simulink model "lab3Koshi"
settings: Solver=ode45  StartTime=0.0  StopTime=100  RelTol=1e-3
libraries: simulink x2
settings Model: Creator=Шландаков  LastModifiedBy=Mihail
settings DataIOCC: LimitDataPoints=on  SaveFormat=Array  ReturnWorkspaceOutputs=off
settings OptimizationCC: LifeSpan=inf  SimCompilerOptimization=Off
settings DebuggingCC: UnderspecifiedInitializationDetection=Classic  MergeDetectMultiDrivingBlocksExec=none  SolverPrmCheckMsg=warning  MultiTaskDSMMsg=warning  MultiTaskCondExecSysMsg=none  FcnCallInpInsideContextMsg=Enable All  FrameProcessingCompatibilityMsg=warning  StateNameClashWarn=warning  StrictBusMsg=None  SFUnexpectedBacktrackingDiag=warning  SFNoUnconditionalDefaultTransitionDiag=warning
settings HardwareCC: ProdBitPerPointer=32  ProdLargestAtomicFloat=None  ProdIntDivRoundTo=Undefined  ProdEndianess=Unspecified  ProdWordSize=32  ProdHWDeviceType=32-bit Generic
settings ModelReferenceCC: PropagateSignalLabelsOutOfModel=off
settings SFSimCC: SimUseLocalCustomCode=off
settings RTWCC: RTWUseLocalCustomCode=off  IncludeERTFirstTime=on  RTWCompilerOptimization=Off
settings GRTTargetCC: CodeReplacementLibrary=ANSI_C  GeneratePreprocessorConditionals=Disable all  CPPClassGenCompliant=off

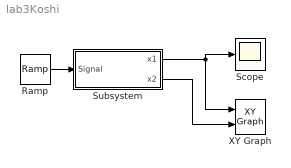
== system lab3Koshi ==
  Ramp : simulink/Sources/Ramp  slope=1  start=0  X0=1
  Scope : Scope
      settings: TimeRange=5  YMin=0  YMax=1000000
  Subsystem : Subsystem  mask{a11=0, a12=1, a21=-1, a22=-2, f1=0, f2=u*(exp(-u)-cos(u)), init1=-1/2, init2=1/2}
      mask prompts: f1 "F1(x)"; f2 "F2(x)"; init1 "Initial (x1(0))"; init2 "Initial (x2(0))"
  XY Graph : simulink/Sinks/XY Graph  xmin=-50  xmax=50  ymin=-50  ymax=50  st=0.1
  wires:
  Subsystem/1(x1) -> Scope/1, XY Graph/1
  Ramp/1 -> Subsystem/1(Signal)
  Subsystem/2(x2) -> XY Graph/2

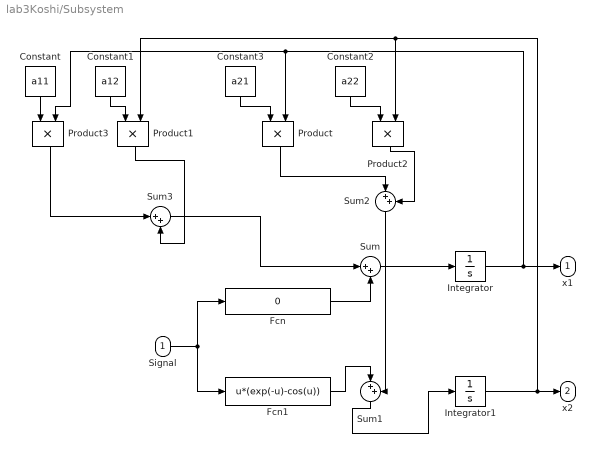
== system lab3Koshi/Subsystem ==
  Signal : Inport
  Constant : Constant  Value=a11
  Constant1 : Constant  Value=a12
  Constant2 : Constant  Value=a22
  Constant3 : Constant  Value=a21
  Fcn : Fcn  Expr=0
  Fcn1 : Fcn  Expr=u*(exp(-u)-cos(u))
  Integrator : Integrator  InitialCondition=init1
  Integrator1 : Integrator  InitialCondition=init2
  Product{,1..3} (4 alike) : Product
  Sum{,1..3} (4 alike) : Sum  Inputs=|++
  x1 : Outport
  x2 : Outport  Port=2
  wires:
  Signal/1 -> Fcn1/1, Fcn/1
  Fcn/1 -> Sum/2
  Fcn1/1 -> Sum1/1
  Sum/1 -> Integrator/1
  Sum1/1 -> Integrator1/1
  Integrator1/1 -> Product1/2, Product2/2, x2/1
  Integrator/1 -> Product3/2, Product/2, x1/1
  Constant2/1 -> Product2/1
  Constant3/1 -> Product/1
  Product/1 -> Sum2/1
  Product2/1 -> Sum2/2
  Sum2/1 -> Sum1/2
  Constant/1 -> Product3/1
  Constant1/1 -> Product1/1
  Product1/1 -> Sum3/2
  Product3/1 -> Sum3/1
  Sum3/1 -> Sum/1
